simulink library "components_lib"  (Simulink 6.2)
undefined symbols (not defined in the file): A_ang_c, A_att_c, A_est, A_kalman, albedo_onboard_wrapper, B_ang_c, B_att_c, B_est, B_kalman, C_ang_c, C_att_c, C_est, C_i, C_kalman, C_p, Cd, D_ang_c, D_att_c, D_est, D_kalman, Dim, DiscIntNeverNeededParam, Hr, Hs, inerti, Ki, Kr, Ks, magnitude, otoquest, otoquest_with_pro, qmethod, rho, sat_temp_start, ss_proj3, sun_emu_angles2currents, sun_emu_vec2angles, Ts, vector_projection_onto_plane, w_mw_i, w_mw_init, zenith2ref
libraries: components_lib x163, simulink x44, albedo_lib x4, Accessories_lib x3, simulink_extras x2, discrete_bdot_filter x1
(part 2 of 5)

== system components_lib/Disturbances/Gravity ==
  R_m(I) : Inport  Port=1  LatchInput=off
  R_s(I) : Inport  Port=2  LatchInput=off
  R_sc(I) : Inport  Port=3  LatchInput=off
  I(C) : Inport  Port=4  LatchInput=off
  "q(I -> S)" : Inport  Port=5  LatchInput=off
  q(C->S) : Inport  Port=6  LatchInput=off
  M_sat : Inport  Port=7  LatchInput=off
  Gain : Gain  Gain=-1  SaturateOnIntegerOverflow=on
  Gravity Gradient Torque : Subsystem
  Gravity Moon : Subsystem
  Gravity Sun : Subsystem
  Product : Product  SaturateOnIntegerOverflow=on
  Sum : Sum  Inputs=+++  SaturateOnIntegerOverflow=on
  Sum1 : Sum  Inputs=|+-  SaturateOnIntegerOverflow=on
  Sum2 : Sum  Inputs=|+-  SaturateOnIntegerOverflow=on
  Zonal Harmonics  Earth : Subsystem
  N_gr(S) : Outport
  F_gr(I) : Outport  Port=2
  wires:
  Gain/1 -> Product/1
  Gravity Sun/1(F_s(I)) -> Sum/2
  Gravity Moon/1(F_m(I)) -> Sum/1
  Sum1/1 -> Gravity Moon/1(R_m_sat(I))
  Sum2/1 -> Gravity Sun/2(R_s_sat(I))
  R_s(I)/1 -> Sum2/1
  R_m(I)/1 -> Sum1/1
  Product/1 -> Sum/3
  Zonal Harmonics  Earth/1(grad(U_zonal(I))) -> Product/2
  Sum/1 -> F_gr(I)/1
  M_sat/1 -> Gain/1, Gravity Sun/1(M_sat), Gravity Moon/2(M_sat)
  Gravity Gradient Torque/1(N_gr(S)) -> N_gr(S)/1
  "q(I -> S)"/1 -> Gravity Gradient Torque/4(q(I->S))
  q(C->S)/1 -> Gravity Gradient Torque/3(q(C->S))
  I(C)/1 -> Gravity Gradient Torque/2(I(C))
  R_sc(I)/1 -> Sum1/2, Sum2/2, Zonal Harmonics  Earth/1(R_sat(I)), Gravity Gradient Torque/1(R_sc(I))

== system components_lib/Disturbances/Magnetic residual disturbance ==
  "Magnetic electronics dipole, d in(S)" : Inport  Port=1  LatchInput=off
  Attitude q(I->S) : Inport  Port=2  LatchInput=off
  Earth rotation q(I->E) : Inport  Port=3  LatchInput=off
  Magnetic field B(E) : Inport  Port=4  LatchInput=off
  Magnetic field E->S : Subsystem
  cross product : Stateflow chart
  N_mres(S) : Outport
  wires:
  "Magnetic electronics dipole, d in(S)"/1 -> cross product/1(u)
  Magnetic field E->S/1(B(S)) -> cross product/2(v)
  cross product/1(y) -> N_mres(S)/1
  Earth rotation q(I->E)/1 -> Magnetic field E->S/2(q(I->E))
  Magnetic field B(E)/1 -> Magnetic field E->S/3(B(E))
  Attitude q(I->S)/1 -> Magnetic field E->S/1(q(I->S))

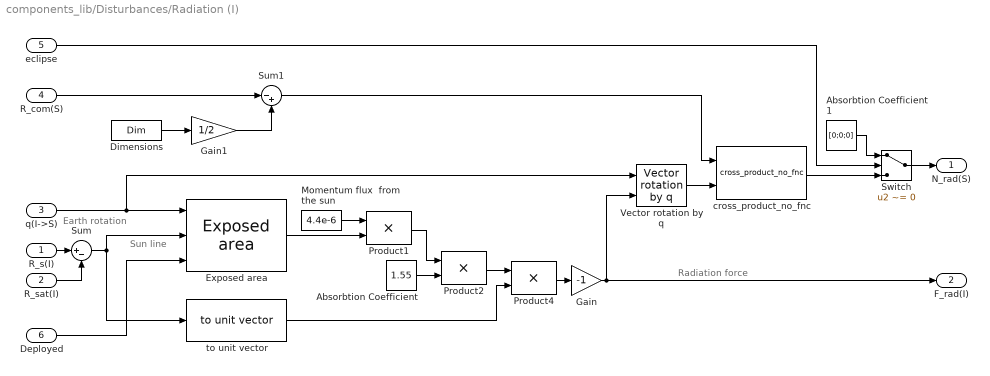
== system components_lib/Disturbances/Radiation (I) ==
  note: Sun line
  note: Earth rotation
  note: Radiation force
  R_s(I) : Inport  Port=1  LatchInput=off
  R_sat(I) : Inport  Port=2  LatchInput=off
  q(I->S) : Inport  Port=3  LatchInput=off
  R_com(S) : Inport  Port=4  LatchInput=off
  eclipse : Inport  Port=5  LatchInput=off
  Deployed : Inport  Port=6  LatchInput=off
  Absorbtion Coefficient : Constant  Value=1.55
  Absorbtion Coefficient1 : Constant  Value=[0;0;0]
  Dimensions : Constant  Value=Dim
  Exposed area : components_lib/Disturbances/Exposed area  dim_sat_area=Dim  dim_sat_array=[-0.30,-0.30]
  Gain : Gain  Gain=-1  SaturateOnIntegerOverflow=on
  Gain1 : Gain  Gain=1/2  SaturateOnIntegerOverflow=on
  Momentum flux  from the sun : Constant  Value=4.4e-6
  Product1 : Product  SaturateOnIntegerOverflow=on
  Product2 : Product  SaturateOnIntegerOverflow=on
  Product4 : Product  SaturateOnIntegerOverflow=on
  Sum : Sum  Inputs=|+-  SaturateOnIntegerOverflow=on
  Sum1 : Sum  Inputs=|-+
  Switch : Switch  Criteria=u2 ~= 0
  Vector rotation by q : components_lib/Math utilities/Quaternion operations/Vector rotation by q
  cross_product_no_fnc : components_lib/Math utilities/Vector operations/cross_product_no_fnc
  to unit vector : components_lib/Math utilities/Vector operations/to unit vector
  N_rad(S) : Outport
  F_rad(I) : Outport  Port=2
  wires:
  Absorbtion Coefficient1/1 -> Switch/1
  Switch/1 -> N_rad(S)/1
  R_s(I)/1 -> Sum/1
  R_sat(I)/1 -> Sum/2
  q(I->S)/1 -> Vector rotation by q/1, Exposed area/1
  Sum/1 -> to unit vector/1, Exposed area/2
  Product1/1 -> Product2/1
  Absorbtion Coefficient/1 -> Product2/2
  Product2/1 -> Product4/1
  to unit vector/1 -> Product4/2
  Product4/1 -> Gain/1
  Gain/1 -> F_rad(I)/1, Vector rotation by q/2
  Vector rotation by q/1 -> cross_product_no_fnc/2
  Exposed area/1 -> Product1/2
  Momentum flux  from the sun/1 -> Product1/1
  cross_product_no_fnc/1 -> Switch/3
  eclipse/1 -> Switch/2
  Dimensions/1 -> Gain1/1
  R_com(S)/1 -> Sum1/1
  Gain1/1 -> Sum1/2
  Sum1/1 -> cross_product_no_fnc/1
  Deployed/1 -> Exposed area/3

== system components_lib/Dynamics and Kinematics/Spacecraft Dynamics ==
  Initial angular velocity W_i(S) : Inport  Port=1  LatchInput=off
  Initial attitude q(I->S) : Inport  Port=2  LatchInput=off
  Controller frame  q(S->C) : Inport  Port=3  LatchInput=off
  Spacecraft Inertia I(C) : Inport  Port=4  LatchInput=off
  N_mt(S) : Inport  Port=5  LatchInput=off
  N_mw(S) : Inport  Port=6  LatchInput=off
  H_mw(S) : Inport  Port=7  LatchInput=off
  Disturbance N_dist(S) : Inport  Port=8  LatchInput=off
  deployed : Inport  Port=9  LatchInput=off
  Inertia deployed I_d(C) : Inport  Port=10  LatchInput=off
  Reverse quaternion rotation : components_lib/Math utilities/Quaternion operations/Reverse quaternion rotation
  Rotation of q1 by q1 : components_lib/Math utilities/Quaternion operations/Rotation of q1 by q2
  Rotation of q1 by q2 : components_lib/Math utilities/Quaternion operations/Rotation of q1 by q2
  Sum : Sum  Inputs=+++  SaturateOnIntegerOverflow=on
  Switch : Switch  Criteria=u2 > Threshold
  Vector rotation by q{,1..3} (4 alike) : components_lib/Math utilities/Vector operations/Vector rotation by q
  sc-dynamics : S-Function  FunctionName=scdynamics
  w to q : components_lib/Math utilities/Quaternion operations/w to q
  Attitude q(I->S) : Outport
  Angular velocity W(S) : Outport  Port=2
  wires:
  N_mw(S)/1 -> Sum/1
  Disturbance N_dist(S)/1 -> Sum/3
  N_mt(S)/1 -> Sum/2
  Vector rotation by q1/1 -> sc-dynamics/2
  Rotation of q1 by q1/1 -> Attitude q(I->S)/1
  sc-dynamics/1 -> Vector rotation by q3/2, w to q/1
  H_mw(S)/1 -> Vector rotation by q2/2
  w to q/1 -> Rotation of q1 by q1/1
  Rotation of q1 by q2/1 -> w to q/2
  Vector rotation by q3/1 -> Angular velocity W(S)/1
  Reverse quaternion rotation/1 -> Vector rotation by q3/1, Rotation of q1 by q1/2
  Vector rotation by q2/1 -> sc-dynamics/3
  Vector rotation by q/1 -> sc-dynamics/1
  Initial attitude q(I->S)/1 -> Rotation of q1 by q2/1
  Controller frame  q(S->C)/1 -> Vector rotation by q/1, Rotation of q1 by q2/2, Vector rotation by q1/1, Reverse quaternion rotation/1, Vector rotation by q2/1
  Initial angular velocity W_i(S)/1 -> Vector rotation by q/2
  Sum/1 -> Vector rotation by q1/2
  Switch/1 -> sc-dynamics/4
  Inertia deployed I_d(C)/1 -> Switch/1
  Spacecraft Inertia I(C)/1 -> Switch/3
  deployed/1 -> Switch/2

== system components_lib/Math utilities/Quaternion operations ==
  Quarternion error : Subsystem
  Quaternion inverter : Subsystem
  Quaternion mulitiplication : S-Function  FunctionName=qmul
  Reverse quaternion rotation : Subsystem
  Rotation from q1 to q2 : Subsystem
  Rotation of q1 by q2 : Subsystem
  Vector rotation by q : Subsystem
  qmul no func : Subsystem
  quaternion composition : Subsystem
  quaternion decomposition : Subsystem
  quaternion expansion : Subsystem
  quaternion2euler : Subsystem
  w to q : Subsystem
  ||q|| : Subsystem

== system components_lib/Math utilities/Vector operations ==
  Projection of a onto b : Subsystem
  Vector rotation by q : Subsystem
  cross_product : Subsystem
  cross_product_no_fnc : Subsystem
  modulus : Subsystem
  norm : Subsystem
  pow : Subsystem  Description=u^v
  sign : Subsystem
  to unit vector : Subsystem
  vector projection onto plane : Subsystem
  ||V|| : MATLABFcn  MATLABFcn=norm

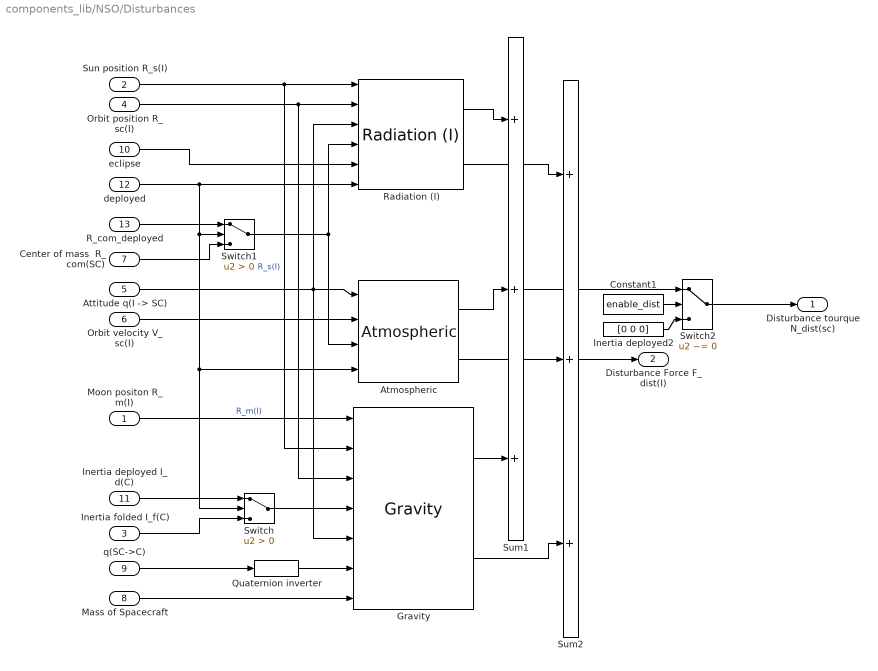
== system components_lib/NSO/Disturbances ==
  Moon positon R_m(I) : Inport  Port=1  LatchInput=off
  Sun position R_s(I) : Inport  Port=2  LatchInput=off
  Inertia folded I_f(C) : Inport  Port=3  LatchInput=off
  Orbit position R_sc(I) : Inport  Port=4  LatchInput=off
  "Attitude q(I -> SC)" : Inport  Port=5  LatchInput=off
  Orbit velocity V_sc(I) : Inport  Port=6  LatchInput=off
  Center of mass  R_com(SC) : Inport  Port=7  LatchInput=off
  "Mass of Spacecraft " : Inport  Port=8  LatchInput=off
  q(SC->C) : Inport  Port=9  LatchInput=off
  eclipse : Inport  Port=10  LatchInput=off
  Inertia deployed I_d(C) : Inport  Port=11  LatchInput=off
  deployed : Inport  Port=12  LatchInput=off
  R_com_deployed : Inport  Port=13  LatchInput=off
  Atmospheric : components_lib/Disturbances/Atmospheric
  Constant1 : Constant  Value=enable_dist
  Gravity : components_lib/Disturbances/Gravity  G=6.673e-11  M_sun=1.98892e30  M_moon=7.36e22  M_earth=5.9742e24
  Inertia deployed2 : Constant  Value=[0 0 0]
  Quaternion inverter : components_lib/Math utilities/Quaternion operations/Quaternion inverter
  Radiation (I) : components_lib/Disturbances/Radiation (I)
  Sum1 : Sum  Inputs=+++  SaturateOnIntegerOverflow=on
  Sum2 : Sum  Inputs=+++  SaturateOnIntegerOverflow=on
  Switch : Switch  Criteria=u2 > Threshold
  Switch1 : Switch  Criteria=u2 > Threshold
  Switch2 : Switch  Criteria=u2 ~= 0
  Disturbance tourque N_dist(sc) : Outport
  Disturbance Force F_dist(I) : Outport  Port=2
  wires:
  deployed/1 -> Radiation (I)/6, Atmospheric/4, Switch/2, Switch1/2
  Switch/1 -> Gravity/4
  Inertia deployed I_d(C)/1 -> Switch/1
  Inertia folded I_f(C)/1 -> Switch/3
  eclipse/1 -> Radiation (I)/5
  Sum2/1 -> Disturbance Force F_dist(I)/1
  Sum1/1 -> Switch2/1
  Gravity/2 -> Sum2/3
  Atmospheric/2 -> Sum2/2
  Radiation (I)/2 -> Sum2/1
  Gravity/1 -> Sum1/3
  Atmospheric/1 -> Sum1/2
  Radiation (I)/1 -> Sum1/1
  Orbit velocity V_sc(I)/1 -> Atmospheric/2
  Orbit position R_sc(I)/1 -> Radiation (I)/2, Gravity/3
  "Attitude q(I -> SC)"/1 -> Gravity/5, Radiation (I)/3, Atmospheric/1
  Sun position R_s(I)/1 -> Radiation (I)/1, Gravity/2  "R_s(I)"
  Moon positon R_m(I)/1 -> Gravity/1  "R_m(I)"
  "Mass of Spacecraft "/1 -> Gravity/7
  Quaternion inverter/1 -> Gravity/6
  q(SC->C)/1 -> Quaternion inverter/1
  Center of mass  R_com(SC)/1 -> Switch1/3
  R_com_deployed/1 -> Switch1/1
  Switch1/1 -> Radiation (I)/4, Atmospheric/3
  Inertia deployed2/1 -> Switch2/3
  Constant1/1 -> Switch2/2
  Switch2/1 -> Disturbance tourque N_dist(sc)/1

== system components_lib/NSO/Spacecraft Dynamics ==
  Initial angular velocity W_i(S) : Inport  Port=1  LatchInput=off
  Initial attitude q(I->S) : Inport  Port=2  LatchInput=off
  Controller frame  q(S->C) : Inport  Port=3  LatchInput=off
  Spacecraft Inertia I(C) : Inport  Port=4  LatchInput=off
  N_mt(S) : Inport  Port=5  LatchInput=off
  N_mw(S) : Inport  Port=6  LatchInput=off
  H_mw(S) : Inport  Port=7  LatchInput=off
  Disturbance N_dist(S) : Inport  Port=8  LatchInput=off
  deployed : Inport  Port=9  LatchInput=off
  Inertia deployed I_d(C) : Inport  Port=10  LatchInput=off
  Reverse quaternion rotation : components_lib/Math utilities/Quaternion operations/Reverse quaternion rotation
  Rotation of q1 by q1 : components_lib/Math utilities/Quaternion operations/Rotation of q1 by q2
  Rotation of q1 by q2 : components_lib/Math utilities/Quaternion operations/Rotation of q1 by q2
  Sum : Sum  Inputs=-++  SaturateOnIntegerOverflow=on
  Switch : Switch  Criteria=u2 > Threshold
  Vector rotation by q{,1..3} (4 alike) : components_lib/Math utilities/Vector operations/Vector rotation by q
  sc-dynamics : S-Function  FunctionName=scdynamics
  w to q : components_lib/Math utilities/Quaternion operations/w to q
  Attitude q(I->S) : Outport
  Angular velocity W(S) : Outport  Port=2
  wires:
  N_mw(S)/1 -> Sum/1
  Disturbance N_dist(S)/1 -> Sum/3
  N_mt(S)/1 -> Sum/2
  Vector rotation by q1/1 -> sc-dynamics/2
  Rotation of q1 by q1/1 -> Attitude q(I->S)/1
  sc-dynamics/1 -> Vector rotation by q3/2, w to q/1
  H_mw(S)/1 -> Vector rotation by q2/2
  w to q/1 -> Rotation of q1 by q1/1
  Rotation of q1 by q2/1 -> w to q/2
  Vector rotation by q3/1 -> Angular velocity W(S)/1
  Reverse quaternion rotation/1 -> Vector rotation by q3/1, Rotation of q1 by q1/2
  Vector rotation by q2/1 -> sc-dynamics/3
  Vector rotation by q/1 -> sc-dynamics/1
  Initial attitude q(I->S)/1 -> Rotation of q1 by q2/1
  Controller frame  q(S->C)/1 -> Vector rotation by q/1, Rotation of q1 by q2/2, Vector rotation by q1/1, Reverse quaternion rotation/1, Vector rotation by q2/1
  Initial angular velocity W_i(S)/1 -> Vector rotation by q/2
  Sum/1 -> Vector rotation by q1/2
  Switch/1 -> sc-dynamics/4
  Inertia deployed I_d(C)/1 -> Switch/1
  Spacecraft Inertia I(C)/1 -> Switch/3
  deployed/1 -> Switch/2

== system components_lib/Orbit and Ephemeris/(IGRF) Magnetic field ==
  Spacecraft position R_sc(I) : Inport  Port=1  LatchInput=off
  Earth rotation q(I->E) : Inport  Port=2  LatchInput=off
  Enable : EnablePort
  Magnetic field model : components_lib/Orbit and Ephemeris/Magnetic field model
  T->Gauss : Gain  Gain=1e4  SaturateOnIntegerOverflow=on
  Vector rotation by q : components_lib/Math utilities/Vector operations/Vector rotation by q
  Magnetic field vector B(E) : Outport
  wires:
  T->Gauss/1 -> Magnetic field vector B(E)/1
  Magnetic field model/1 -> T->Gauss/1  "B(I / E)"
  Vector rotation by q/1 -> Magnetic field model/1
  Earth rotation q(I->E)/1 -> Vector rotation by q/1
  Spacecraft position R_sc(I)/1 -> Vector rotation by q/2

== system components_lib/Orbit and Ephemeris/Albedo ==
  Sunlight vector(I) : Inport  Port=1  LatchInput=off
  Nadir vector (I) : Inport  Port=2  LatchInput=off
  q(I>E) : Inport  Port=3  LatchInput=off
  Enable : EnablePort
  Earth Albedo Model : albedo_lib/Earth Albedo Model  eprdata=load('lib/space_environment_emulation/albedo/toolbox/epr_data/2003/ga030101-031231')  redfac=1  Ts=10  enable=on
  Vector rotation by q1 : components_lib/Math utilities/Vector operations/Vector rotation by q
  Vector rotation by q2 : components_lib/Math utilities/Vector operations/Vector rotation by q
  Reflectivity matrix : Outport
  wires:
  Sunlight vector(I)/1 -> Vector rotation by q2/2
  q(I>E)/1 -> Vector rotation by q2/1, Vector rotation by q1/1
  Nadir vector (I)/1 -> Vector rotation by q1/2
  Earth Albedo Model/1 -> Reflectivity matrix/1
  Vector rotation by q2/1 -> Earth Albedo Model/2
  Vector rotation by q1/1 -> Earth Albedo Model/1

== system components_lib/Orbit and Ephemeris/Albedo emulation model ==
  Sunlight vector(I) : Inport  Port=1  LatchInput=off
  Nadir vector (I) : Inport  Port=2  LatchInput=off
  q(I>E) : Inport  Port=3  LatchInput=off
  Earth Albedo Model1 : albedo_lib/Earth Albedo Model  eprdata=mean_epr  redfac=1  Ts=60  enable=on
  Vector rotation by q1 : components_lib/Math utilities/Vector operations/Vector rotation by q
  Vector rotation by q2 : components_lib/Math utilities/Vector operations/Vector rotation by q
  Reflectivity matrix : Outport
  wires:
  Vector rotation by q1/1 -> Earth Albedo Model1/1
  Vector rotation by q2/1 -> Earth Albedo Model1/2
  Earth Albedo Model1/1 -> Reflectivity matrix/1
  Nadir vector (I)/1 -> Vector rotation by q1/2
  q(I>E)/1 -> Vector rotation by q1/1, Vector rotation by q2/1
  Sunlight vector(I)/1 -> Vector rotation by q2/2

== system components_lib/Orbit and Ephemeris/Eclipse model ==
  note: theta_e
  Sun vector (I) : Inport  Port=1  LatchInput=off
  Satellite (I) : Inport  Port=2  LatchInput=off
  Constant : Constant  Value=pi
  Divide : Product  Inputs=*/  OutScaling=2^-10
  Dot Product : simulink/Math Operations/Dot Product  InputSameDT=on  OutDataType=sfix(16)  OutScaling=2^-10  DoSatur=off
  Dot Product1 : simulink/Math Operations/Dot Product  InputSameDT=on  OutDataType=sfix(16)  OutScaling=2^-10  DoSatur=off
  Earth radius : Constant  Value=r_e
  False : Constant  Value=0
  Manual Switch : simulink/Signal Routing/Manual Switch  sw=0  action=0
  Math Function : Math  Operator=sqrt  SaturateOnIntegerOverflow=on
  Max angle : Constant  Value=theta_e/180*pi
  Satellite unit vector : components_lib/Math utilities/Vector operations/to unit vector
  Sum : Sum  Orientation=down  Inputs=-+|
  Sum1 : Sum  Inputs=+-|
  Sun unit vector : components_lib/Math utilities/Vector operations/to unit vector
  Switch : Switch
  Trigonometric Function : Trigonometry  Operator=asin
  Trigonometric Function1 : Trigonometry  Operator=acos
  True : Constant
  "Eclipse: 1 = true, 0 = false" : Outport  PortDimensions=1
  wires:
  Sun vector (I)/1 -> Sun unit vector/1
  Satellite (I)/1 -> Satellite unit vector/1, Dot Product1/1, Dot Product1/2
  Sun unit vector/1 -> Dot Product/1
  Satellite unit vector/1 -> Dot Product/2
  Dot Product/1 -> Trigonometric Function1/1
  Earth radius/1 -> Divide/1
  Math Function/1 -> Divide/2
  Divide/1 -> Trigonometric Function/1
  Trigonometric Function1/1 -> Sum/1
  Constant/1 -> Sum/2
  Sum/1 -> Sum1/1  "theta"
  Sum1/1 -> Switch/2
  True/1 -> Switch/3
  False/1 -> Switch/1
  Switch/1 -> "Eclipse: 1 = true, 0 = false"/1
  Manual Switch/1 -> Sum1/2
  Trigonometric Function/1 -> Manual Switch/2
  Max angle/1 -> Manual Switch/1
  Dot Product1/1 -> Math Function/1

== system components_lib/Orbit and Ephemeris/Ephemeris ==
  Time t(JD) : Inport  Port=1  LatchInput=off
  ECEF : Subsystem
  Moon Position : Subsystem
  Sun Position : Subsystem
  Moon position R_m(I) : Outport
  Sun Position R_s(I) : Outport  Port=2
  Earth Rotation q(I->E) : Outport  Port=3
  wires:
  ECEF/1(q(I->E)) -> Earth Rotation q(I->E)/1  "q(I -> E)"
  Time t(JD)/1 -> Moon Position/1(t(JD)1), Sun Position/1(t(JD)), ECEF/1(t(JD))  "t"
  Moon Position/1(R_m(I)) -> Moon position R_m(I)/1  "R_m(I)"
  Sun Position/1(R_s(I)) -> Sun Position R_s(I)/1  "R_s(I)"

== system components_lib/Orbit and Ephemeris/Magnetic field model ==
  R_sc(E) : Inport  Port=1  LatchInput=off
  S-Function : S-Function  FunctionName=igrfS  Parameters=2002,10
  B(E) : Outport
  wires:
  R_sc(E)/1 -> S-Function/1
  S-Function/1 -> B(E)/1

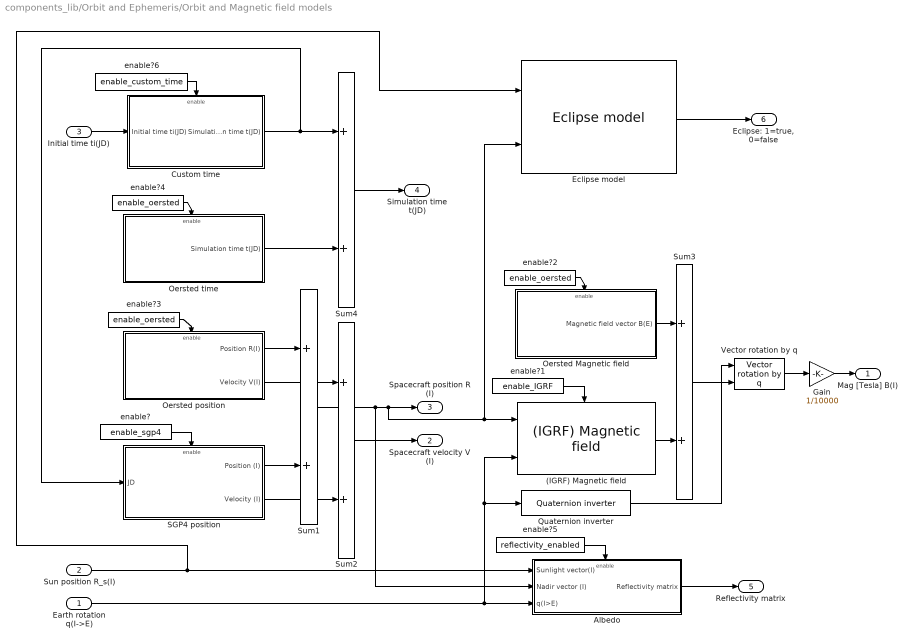
== system components_lib/Orbit and Ephemeris/Orbit and Magnetic field models ==
  Earth rotation q(I->E) : Inport  Port=1  LatchInput=off
  Sun position R_s(I) : Inport  Port=2  LatchInput=off
  Initial time ti(JD) : Inport  Port=3  LatchInput=off
  (IGRF) Magnetic field : components_lib/Orbit and Ephemeris/(IGRF) Magnetic field
  Albedo : Subsystem  AncestorBlock=components_lib/Orbit and Ephemeris/Albedo  TreatAsAtomicUnit=on
  Custom time : Subsystem  TreatAsAtomicUnit=on
  Eclipse model : components_lib/Orbit and Ephemeris/Eclipse model  r_e=6371010  theta_e=65
  Gain : Gain  Gain=1/10000
  Oersted Magnetic field : Subsystem  TreatAsAtomicUnit=on
  Oersted position : Subsystem  TreatAsAtomicUnit=on
  Oersted time : Subsystem  TreatAsAtomicUnit=on
  Quaternion inverter : components_lib/Math utilities/Quaternion operations/Quaternion inverter
  SGP4 position : Subsystem  TreatAsAtomicUnit=on
  Sum{1..4} (4 alike) : Sum
  Vector rotation by q : components_lib/Math utilities/Quaternion operations/Vector rotation by q
  enable? : Constant  Value=enable_sgp4
  enable?1 : Constant  Value=enable_IGRF
  enable?2 : Constant  Value=enable_oersted
  enable?3 : Constant  Value=enable_oersted
  enable?4 : Constant  Value=enable_oersted
  enable?5 : Constant  Value=reflectivity_enabled
  enable?6 : Constant  Value=enable_custom_time
  Mag [Tesla] B(I) : Outport
  Spacecraft velocity V (I) : Outport  Port=2
  Spacecraft position R (I) : Outport  Port=3
  Simulation time t(JD) : Outport  Port=4
  Reflectivity matrix : Outport  Port=5
  "Eclipse: 1=true, 0=false" : Outport  Port=6  PortDimensions=1
  wires:
  Gain/1 -> Mag [Tesla] B(I)/1
  Sum3/1 -> Vector rotation by q/2
  (IGRF) Magnetic field/1 -> Sum3/2
  Oersted Magnetic field/1(Magnetic field vector B(E)) -> Sum3/1
  Sum2/1 -> Spacecraft velocity V (I)/1
  Sum1/1 -> Spacecraft position R (I)/1, Eclipse model/2, (IGRF) Magnetic field/1, Albedo/2(Nadir vector (I))
  SGP4 position/2(Velocity (I)) -> Sum2/2
  Oersted position/2(Velocity V(I)) -> Sum2/1
  SGP4 position/1(Position (I)) -> Sum1/2
  Oersted position/1(Position R(I)) -> Sum1/1
  enable?4/1 -> Oersted time/Enable
  enable?/1 -> SGP4 position/Enable
  Earth rotation q(I->E)/1 -> Quaternion inverter/1, (IGRF) Magnetic field/2, Albedo/3(q(I>E))
  Sun position R_s(I)/1 -> Eclipse model/1, Albedo/1(Sunlight vector(I))
  Albedo/1(Reflectivity matrix) -> Reflectivity matrix/1
  enable?3/1 -> Oersted position/Enable
  Initial time ti(JD)/1 -> Custom time/1(Initial time ti(JD))
  Oersted time/1(Simulation time t(JD)) -> Sum4/2
  Custom time/1(Simulation time t(JD)) -> Sum4/1, SGP4 position/1(JD)
  Sum4/1 -> Simulation time t(JD)/1
  enable?6/1 -> Custom time/Enable
  Quaternion inverter/1 -> Vector rotation by q/1
  Vector rotation by q/1 -> Gain/1
  enable?1/1 -> (IGRF) Magnetic field/Enable
  enable?2/1 -> Oersted Magnetic field/Enable
  enable?5/1 -> Albedo/Enable
  Eclipse model/1 -> "Eclipse: 1=true, 0=false"/1

== system components_lib/Other model utilities/AAUSAT-II Animation ==
  SC position : Inport  Port=1  LatchInput=off
  SC quaternion : Inport  Port=2  LatchInput=off
  SC veloc : Inport  Port=3  LatchInput=off
  sun vector(I) : Inport  Port=4  LatchInput=off
  Earth rotation : Inport  Port=5  LatchInput=off
  Mux3 : Mux  Inputs=5
  S-Function : S-Function  FunctionName=aausatanim  Parameters=Config
  wires:
  Mux3/1 -> S-Function/1
  SC position/1 -> Mux3/1
  SC quaternion/1 -> Mux3/2
  sun vector(I)/1 -> Mux3/4
  Earth rotation/1 -> Mux3/5
  SC veloc/1 -> Mux3/3

== system components_lib/Sensor Emulation/Emulation of gyros ==
  W(S) [rad/s] : Inport  Port=1  LatchInput=off
  Temperature [K] : Inport  Port=2  LatchInput=off
  Amplification and ADC : Subsystem
  Demux : Demux  Outputs=3
  Demux1 : Demux  Outputs=3
  Gain : Gain  Gain=-1
  Gyro sensor block : Subsystem
  Mux : Mux  Inputs=6
  V_ADC [mV] : Outport
  wires:
  Amplification and ADC/1(V_discrete) -> V_ADC [mV]/1
  Demux/3 -> Mux/6
  Demux/2 -> Mux/5
  Demux/1 -> Mux/4
  Demux1/3 -> Mux/3
  Demux1/2 -> Mux/2
  Demux1/1 -> Mux/1
  Gain/1 -> Demux/1
  W(S) [rad/s]/1 -> Gain/1, Demux1/1
  Mux/1 -> Gyro sensor block/1(W(S) [rad/s])
  Temperature [K]/1 -> Gyro sensor block/2(Temperature [K])
  Gyro sensor block/1(W_sens(S) [mV]) -> Amplification and ADC/1(V_cont)

== system components_lib/Sensor Emulation/Emulation of magnetometer ==
  B(I) : Inport  Port=1  LatchInput=off
  q(I->S) : Inport  Port=2  LatchInput=off
  Temperature  [K] : Inport  Port=3  LatchInput=off
  Amplification and ADC : Subsystem
  magnetometer sensor block : Subsystem
  V_ADC [mV] : Outport
  wires:
  magnetometer sensor block/1(Voltage  [mV]) -> Amplification and ADC/1(V_cont)
  Amplification and ADC/1(V_discrete) -> V_ADC [mV]/1
  B(I)/1 -> magnetometer sensor block/1(B(I))
  q(I->S)/1 -> magnetometer sensor block/2(q(I->S))
  Temperature  [K]/1 -> magnetometer sensor block/3(Temperature  [K])

== system components_lib/Sensor Emulation/Emulation of temperature sensors ==
  Band-Limited White Noise : simulink/Sources/Band-Limited White Noise  Cov=1e-9  Ts=1  seed=33232
  Constant : Constant  Value=sat_temp_start
  Sum : Sum  Inputs=|++
  Temperature_meas [mV] : Outport
  Temperature [K] : Outport  Port=2
  wires:
  Sum/1 -> Temperature_meas [mV]/1
  Constant/1 -> Sum/1, Temperature [K]/1
  Band-Limited White Noise/1 -> Sum/2

== system components_lib/Sensor Emulation/Sensor Emulation ==
  Attitude q(I->S) : Inport  Port=1  LatchInput=off
  Mag. field B(I) : Inport  Port=2  LatchInput=off
  Sun pos. R_s(I) : Inport  Port=3  LatchInput=off
  Earth rot. q(I->E) : Inport  Port=4  LatchInput=off
  Ang. vel. W(S) : Inport  Port=5  LatchInput=off
  S/C pos. R_sa(I) : Inport  Port=6  LatchInput=off
  Reflectivity matrix : Inport  Port=7  LatchInput=off
  Eclipse sim : Inport  Port=8  LatchInput=off
  Enable : EnablePort
  Emulation of gyros : components_lib/Sensor Emulation/Emulation of gyros  scale_model=[859.4 859.4 859.4 859.4 859.4 859.4]  offset_model=[2500 2500 2500 2500 2500 2500]  e_bias=[0.0012 0.0012 0.0012 0.0012 0.0012 0.0012]  e_align=[1 1 1 1 1 1]  e_scale=[0.1 0.1 0.1 0.1 0.1 0.1]  e_noise=[0.0035 0.0035 0.0035 0.0035 0.0035 0.0035]*1e-6  e_noise_seed=[23341 43534 43433 22299 32478 21932]  e_drift_scale_model=[0.075 0.075 0.075 0.075 0.075 0.075]  e_drift_offset_model=[0.012 0.012 0.012 0.012 0.012 0.012]  op_amp_gain=[10 10 10 10 10 10]  op_amp_offset=[2500 2500 2500 2500 2500 2500]
  Emulation of magnetometer : components_lib/Sensor Emulation/Emulation of magnetometer  v_supply_model=5  sens_model=[1 1 1]  e_drift_sens_model=[-3000 -3000 -3000]  e_scale=[0.05 0.05 0.05]  e_align=1*0  e_orth=1*0  e_noise=[32 32 32]*1e-6*0  e_noise_seed=[23341 43534 43433]  op_amp_gain=[500 500 500]  op_amp_offset=[2500 2500 2500]
  Emulation of temperature sensors : components_lib/Sensor Emulation/Emulation of temperature sensors
  Sun sensors : components_lib/Sensor Emulation/Sun sensors  sun_flux=1366.9  alpha_align=[1 1 1 1 2 2]*0  temp_drift=0.00233  sigma_noise=0.0000014*0  noise_seed=[0.0000008 0.0000011 0.0000004 0.0000005 0.0000000 0.0000002]*0  op_amp_gain=1  op_amp_offset=0
  Magnotometer (S)  V_ADC [mV] : Outport
  Gyros  (S) V_ADC [mV] : Outport  Port=2
  Sun sensors (S)  [mA] : Outport  Port=3
  Temperature (S) V_ADC [mV] : Outport  Port=4
  wires:
  Mag. field B(I)/1 -> Emulation of magnetometer/1
  Attitude q(I->S)/1 -> Emulation of magnetometer/2, Sun sensors/4
  Earth rot. q(I->E)/1 -> Sun sensors/5
  Emulation of magnetometer/1 -> Magnotometer (S)  V_ADC [mV]/1
  Ang. vel. W(S)/1 -> Emulation of gyros/1
  Emulation of gyros/1 -> Gyros  (S) V_ADC [mV]/1
  S/C pos. R_sa(I)/1 -> Sun sensors/2
  Sun pos. R_s(I)/1 -> Sun sensors/1
  Sun sensors/1 -> Sun sensors (S)  [mA]/1
  Reflectivity matrix/1 -> Sun sensors/3
  Emulation of temperature sensors/1 -> Temperature (S) V_ADC [mV]/1
  Emulation of temperature sensors/2 -> Emulation of magnetometer/3, Sun sensors/6, Emulation of gyros/2
  Eclipse sim/1 -> Sun sensors/7

== system components_lib/Sensor Emulation/Sun sensors ==
  Sun pos. R_s(I) : Inport  Port=1  LatchInput=off
  S/C pos. R_sa(I) : Inport  Port=2  LatchInput=off
  Reflectivity matrix : Inport  Port=3  LatchInput=off
  q(I->S) : Inport  Port=4  LatchInput=off
  q(I->E) : Inport  Port=5  LatchInput=off
  Temperature  [K] : Inport  Port=6  LatchInput=off
  Eclipse sim : Inport  Port=7  LatchInput=off
  Amplification and ADC : Subsystem
  Frame conversion : Subsystem
  q rot : Scope  NumInputPorts=3
      settings: YMin=-3e+10~-5~-5  YMax=1.5e+11~5~5  SaveName=ScopeData5
  sun sensor model : Subsystem
  Sun_currents [mA] : Outport
  wires:
  Eclipse sim/1 -> sun sensor model/6(Eclipse sim)
  Frame conversion/3(q(S->E)) -> sun sensor model/3(q(S->E))
  q(I->E)/1 -> Frame conversion/4(q(I->E))
  sun sensor model/1(Currents [mA]) -> q rot/3, Amplification and ADC/1(Currents [mA])  "currents"
  Reflectivity matrix/1 -> sun sensor model/4(Reflectivity matrix)
  Temperature  [K]/1 -> sun sensor model/5(Temperature  [K])
  Frame conversion/1(Sun pos. R_s(S)) -> q rot/2, sun sensor model/1(Sun position R_s(S))
  Frame conversion/2(Nadir(E)) -> q rot/1, sun sensor model/2(Nadir(E))  "nadir (E)"
  S/C pos. R_sa(I)/1 -> Frame conversion/2(S/C pos. R_sa(I))
  Sun pos. R_s(I)/1 -> Frame conversion/1(Sun pos. R_s(I))
  q(I->S)/1 -> Frame conversion/3(q(I->S))
  Amplification and ADC/1(I_ADC [mA]) -> Sun_currents [mA]/1

== system components_lib/ACS/Controllers/Angular velocity  controller ==
  omega : Inport  Port=1  LatchInput=off
  omega_ref : Inport  Port=2  LatchInput=off
  State-Space : StateSpace  A=A_ang_c  B=B_ang_c  C=C_ang_c  D=D_ang_c
  Sum : Sum  Inputs=|+-
  N_mw : Outport
  wires:
  omega_ref/1 -> Sum/2
  omega/1 -> Sum/1
  State-Space/1 -> N_mw/1
  Sum/1 -> State-Space/1

== system components_lib/ACS/Controllers/Attitude controller ==
  q_att : Inport  Port=1  LatchInput=off
  q_ref : Inport  Port=2  LatchInput=off
  omega : Inport  Port=3  LatchInput=off
  Mux : Mux  Inputs=2
  Quarternion error : components_lib/Math utilities/Quaternion operations/Quarternion error
  Selector : Selector  Elements=[1 2 3]  InputPortWidth=4
  State-Space : StateSpace  A=A_att_c  B=B_att_c  C=C_att_c  D=D_att_c
  omega_ref : Outport
  wires:
  State-Space/1 -> omega_ref/1
  Quarternion error/1 -> Selector/1
  q_att/1 -> Quarternion error/1
  q_ref/1 -> Quarternion error/2
  Selector/1 -> Mux/1
  omega/1 -> Mux/2
  Mux/1 -> State-Space/1

== system components_lib/ACS/Controllers/Attitude controller with integrator ==
  q_att : Inport  Port=1  LatchInput=off
  q_ref : Inport  Port=2  LatchInput=off
  omega : Inport  Port=3  LatchInput=off
  Integrator : Integrator  LimitOutput=on  UpperSaturationLimit=0.01  LowerSaturationLimit=-0.01
  Mux : Mux  Inputs=3
  Quarternion error : components_lib/Math utilities/Quaternion operations/Quarternion error
  Selector : Selector  Elements=[1 2 3]  InputPortWidth=4
  State-Space : StateSpace  A=A_att_c  B=B_att_c  C=C_att_c  D=D_att_c
  omega_ref : Outport
  wires:
  Mux/1 -> State-Space/1
  omega/1 -> Mux/2
  Selector/1 -> Mux/1, Integrator/1
  q_ref/1 -> Quarternion error/2
  q_att/1 -> Quarternion error/1
  Quarternion error/1 -> Selector/1
  State-Space/1 -> omega_ref/1
  Integrator/1 -> Mux/3

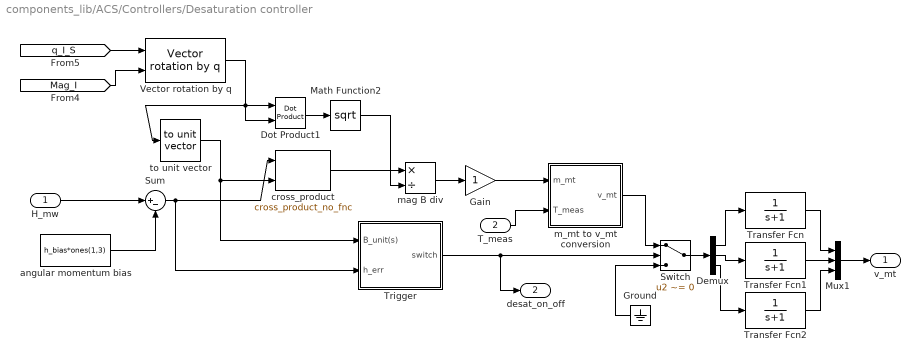
== system components_lib/ACS/Controllers/Desaturation controller ==
  H_mw : Inport  Port=1  LatchInput=off
  T_meas : Inport  Port=2  LatchInput=off
  Demux : Demux  Outputs=3
  Dot Product1 : simulink/Math Operations/Dot Product  InputSameDT=on  OutDataType=sfix(16)  OutScaling=2^-10  DoSatur=off
  Gain : Gain
  Ground : Ground  Orientation=left
  Math Function2 : Math  Operator=sqrt  SaturateOnIntegerOverflow=on
  Mux1 : Mux  Inputs=3
  Sum : Sum  Inputs=|+-
  Switch : Switch  Criteria=u2 ~= 0  Threshold=0.5
  Transfer Fcn : TransferFcn  Denominator=[1 1]
  Transfer Fcn1 : TransferFcn  Denominator=[1 1]
  Transfer Fcn2 : TransferFcn  Denominator=[1 1]
  Trigger : Subsystem
  Vector rotation by q : components_lib/Math utilities/Quaternion operations/Vector rotation by q
  angular momentum bias : Constant  Value=h_bias*ones(1,3)
  cross_product : components_lib/Math utilities/Vector operations/cross_product_no_fnc
  m_mt to v_mt conversion : Subsystem  mask{n_mt=[435 435 865], A_mt=[0.21*0.07 0.21*0.07 0.07*0.07], L_mt=[26.956e-3 26.956e-3 59.256e-3], v_max_mt=5}
      mask prompts: n_mt "Coil winding number [n_x n_y n_z]"; A_mt "Coil area [A_mt_x A_mt_y A_mt_z]"; L_mt "Coil inductance [L_mt_x L_mt_y L_mt_z]"; v_max_mt "Maximum voltage"
  mag B div : Product  Inputs=*/  OutScaling=2^-10
  to unit vector : components_lib/Math utilities/Vector operations/to unit vector
  v_mt : Outport
  desat_on_off : Outport  Port=2
  wires:
  H_mw/1 -> Sum/1
  angular momentum bias/1 -> Sum/2
  [Mag_I] -> Vector rotation by q/2
  [q_I_S] -> Vector rotation by q/1
  Sum/1 -> cross_product/1, Trigger/2(h_err)
  cross_product/1 -> mag B div/1
  Ground/1 -> Switch/3
  T_meas/1 -> m_mt to v_mt conversion/2(T_meas)
  mag B div/1 -> Gain/1
  m_mt to v_mt conversion/1(v_mt) -> Switch/1
  Dot Product1/1 -> Math Function2/1
  Math Function2/1 -> mag B div/2
  Gain/1 -> m_mt to v_mt conversion/1(m_mt)
  Switch/1 -> Demux/1
  Demux/1 -> Transfer Fcn/1
  Demux/2 -> Transfer Fcn1/1
  Demux/3 -> Transfer Fcn2/1
  Transfer Fcn/1 -> Mux1/1
  Transfer Fcn1/1 -> Mux1/2
  Transfer Fcn2/1 -> Mux1/3
  Mux1/1 -> v_mt/1
  Vector rotation by q/1 -> Dot Product1/2, Dot Product1/1, to unit vector/1
  to unit vector/1 -> cross_product/2, Trigger/1(B_unit(s))
  Trigger/1(switch) -> Switch/2, desat_on_off/1

== system components_lib/ACS/Controllers/Detumble controller ==
  q(I->S) : Inport  Port=1  LatchInput=off
  B(I) : Inport  Port=2  LatchInput=off
  Constant : Constant  Value=ctrl
  Continous B-dot controller : Subsystem
  Discrete B-dot controller : Subsystem
  Magnetic field I to S : Subsystem
  Merge : Merge
  Switch Case : SwitchCase  CaseConditions={2,3}  CaseShowDefault=off
  enable/disable continous controller : Subsystem  TreatAsAtomicUnit=on
  enable/disable discrete controller : Subsystem  TreatAsAtomicUnit=on
  m_mt(S) : Outport
  wires:
  Switch Case/1 -> enable/disable continous controller/Action
  enable/disable continous controller/1(Out1) -> Merge/1
  Continous B-dot controller/1(m_mt(S)) -> enable/disable continous controller/1(In1)
  enable/disable discrete controller/1(Out1) -> Merge/2
  Discrete B-dot controller/1(m_mt(s)) -> enable/disable discrete controller/1(In1)
  Merge/1 -> m_mt(S)/1
  Switch Case/2 -> enable/disable discrete controller/Action
  Constant/1 -> Switch Case/1
  Magnetic field I to S/1(B(S)) -> Continous B-dot controller/1(B(S)), Discrete B-dot controller/1(B(S))
  q(I->S)/1 -> Magnetic field I to S/1(q(I->S))
  B(I)/1 -> Magnetic field I to S/2(B(I))

== system components_lib/ACS/Controllers/Estimation of dist Kalman filter ==
  control_torque : Inport  Port=1  LatchInput=off
  omega : Inport  Port=2  LatchInput=off
  Mux : Mux  Inputs=2
  State-Space : StateSpace  A=A_kalman  B=B_kalman  C=C_kalman  D=D_kalman
  estimated disturbance : Outport
  wires:
  omega/1 -> Mux/2
  Mux/1 -> State-Space/1
  control_torque/1 -> Mux/1
  State-Space/1 -> estimated disturbance/1

== system components_lib/ACS/Controllers/Estimation of dist linear filter ==
  control_torque : Inport  Port=1  LatchInput=off
  omega : Inport  Port=2  LatchInput=off
  Mux : Mux  Inputs=2
  State-Space : StateSpace  A=A_est  B=B_est  C=C_est  D=D_est
  estimated disturbance : Outport
  wires:
  State-Space/1 -> estimated disturbance/1
  control_torque/1 -> Mux/1
  Mux/1 -> State-Space/1
  omega/1 -> Mux/2

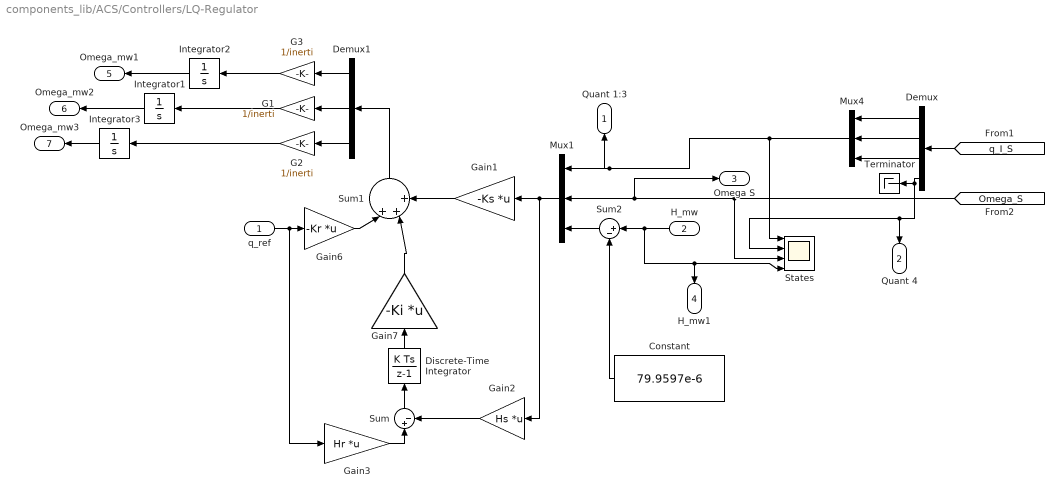
== system components_lib/ACS/Controllers/LQ-Regulator ==
  q_ref : Inport  Port=1  LatchInput=off
  H_mw : Inport  Orientation=left  Port=2  LatchInput=off
  Constant : Constant  Orientation=left  Value=79.9597e-6
  Demux : Demux  Orientation=left
  Demux1 : Demux  Orientation=left  Outputs=3
  Discrete-Time Integrator : DiscreteIntegrator  Orientation=up  SampleTime=Ts  ICPrevOutput=DiscIntNeverNeededParam  ICPrevScaledInput=DiscIntNeverNeededParam
  G1 : Gain  Orientation=left  Gain=1/inerti
  G2 : Gain  Orientation=left  Gain=1/inerti
  G3 : Gain  Orientation=left  Gain=1/inerti
  Gain1 : Gain  Orientation=left  Gain=-Ks  Multiplication=Matrix(K*u)
  Gain2 : Gain  Orientation=left  Gain=Hs  Multiplication=Matrix(K*u)
  Gain3 : Gain  Gain=Hr  Multiplication=Matrix(K*u)
  Gain6 : Gain  Gain=-Kr  Multiplication=Matrix(K*u)
  Gain7 : Gain  Orientation=up  Gain=-Ki  Multiplication=Matrix(K*u)
  Integrator1 : Integrator  Orientation=left  LimitOutput=on  UpperSaturationLimit=576  LowerSaturationLimit=-576
  Integrator2 : Integrator  Orientation=left  LimitOutput=on  UpperSaturationLimit=576  LowerSaturationLimit=-576
  Integrator3 : Integrator  Orientation=left  LimitOutput=on  UpperSaturationLimit=576  LowerSaturationLimit=-576
  Mux1 : Mux  Orientation=left  Inputs=3
  Mux4 : Mux  Orientation=left  Inputs=3
  States : Scope  NumInputPorts=4
      settings: TimeRange=600  YMin=-0.2~0.9225~-0.0125~0  YMax=0.4~0.9475~0.0125~0.00014
  Sum : Sum  Orientation=up  Inputs=|+-
  Sum1 : Sum  Orientation=up  Inputs=|+++
  Sum2 : Sum  Orientation=left  Inputs=|+-
  Terminator : Terminator
  Quant 1:3 : Outport  Orientation=up
  Quant 4 : Outport  Orientation=down  Port=2
  Omega S : Outport  Port=3
  H_mw1 : Outport  Orientation=down  Port=4
  Omega_mw1 : Outport  Orientation=left  Port=5
  Omega_mw2 : Outport  Orientation=left  Port=6
  Omega_mw3 : Outport  Orientation=left  Port=7
  wires:
  Mux1/1 -> Gain1/1, Gain2/1
  Gain2/1 -> Sum/2
  Gain3/1 -> Sum/1
  Sum/1 -> Discrete-Time Integrator/1
  Discrete-Time Integrator/1 -> Gain7/1
  Gain1/1 -> Sum1/3
  Gain7/1 -> Sum1/2
  Gain6/1 -> Sum1/1
  q_ref/1 -> Gain6/1, Gain3/1
  Constant/1 -> Sum2/2
  Sum2/1 -> Mux1/3
  Demux/4 -> Terminator/1, States/2, Quant 4/1
  [q_I_S] -> Demux/1
  Demux/1 -> Mux4/1
  Demux/2 -> Mux4/2
  Demux/3 -> Mux4/3
  [Omega_S] -> States/3, Mux1/2, Omega S/1
  Mux4/1 -> States/1, Mux1/1, Quant 1:3/1
  Sum1/1 -> Demux1/1
  H_mw/1 -> Sum2/1, States/4, H_mw1/1
  G3/1 -> Integrator2/1
  G1/1 -> Integrator1/1
  G2/1 -> Integrator3/1
  Demux1/1 -> G3/1
  Demux1/2 -> G1/1
  Demux1/3 -> G2/1
  Integrator2/1 -> Omega_mw1/1
  Integrator1/1 -> Omega_mw2/1
  Integrator3/1 -> Omega_mw3/1

== system components_lib/ADS/Attitude Determination/EKF using quaternions ==
  q : Inport  Port=1  LatchInput=off
  w : Inport  Port=2  LatchInput=off
  h_mw : Inport  Port=3  LatchInput=off
  N_mt : Inport  Port=4  LatchInput=off
  q0_in : Inport  Port=5  LatchInput=off
  eclipse : Inport  Port=6  LatchInput=off
  Clock : Clock
      settings: Decimation=10
  Demux1 : Demux  Outputs=16
  EKF : MATLABFcn  MATLABFcn=AAUSAT_II_Kalman  OutputDimensions=16  SampleTime=0.1
  Mux1 : Mux  Inputs=3
  Mux2 : Mux  Inputs=8
  Mux3 : Mux
  Mux4 : Mux  Inputs=3
  Mux5 : Mux  Inputs=3
  Step size : Constant  Value=0.1
  q_out : Outport
  w_out : Outport  Port=2
  q_residual : Outport  Port=3
  w_residual : Outport  Port=4
  wires:
  eclipse/1 -> Mux2/8
  q0_in/1 -> Mux2/6
  q/1 -> Mux2/1
  Mux4/1 -> w_out/1
  Mux3/1 -> q_out/1
  N_mt/1 -> Mux2/4
  h_mw/1 -> Mux2/3
  w/1 -> Mux2/2
  Clock/1 -> Mux2/5
  Demux1/4 -> Mux3/4
  Demux1/3 -> Mux3/3
  Demux1/2 -> Mux3/2
  Demux1/1 -> Mux3/1
  Step size/1 -> Mux2/7
  EKF/1 -> Demux1/1
  Mux2/1 -> EKF/1
  Mux1/1 -> q_residual/1
  Mux5/1 -> w_residual/1
  Demux1/8 -> Mux1/1
  Demux1/9 -> Mux1/2
  Demux1/10 -> Mux1/3
  Demux1/5 -> Mux4/1
  Demux1/6 -> Mux4/2
  Demux1/7 -> Mux4/3
  Demux1/11 -> Mux5/1
  Demux1/12 -> Mux5/2
  Demux1/13 -> Mux5/3

== system components_lib/ADS/Attitude Determination/EKF using sun and mag vectors ==
  R_sun(S) : Inport  Port=1  LatchInput=off
  b(S) : Inport  Port=2  LatchInput=off
  w(S) : Inport  Port=3  LatchInput=off
  R_sun(I) : Inport  Port=4  LatchInput=off
  b(I) : Inport  Port=5  LatchInput=off
  h_mw : Inport  Port=6  LatchInput=off
  N_mt : Inport  Port=7  LatchInput=off
  q0 : Inport  Port=8  LatchInput=off
  Eclipse : Inport  Port=9  LatchInput=off
  Clock : Clock
      settings: Decimation=10
  Demux1 : Demux  Outputs=7
  EKF : MATLABFcn  MATLABFcn=AAUSAT_II_Kalman_BS_vectors  OutputDimensions=7  SampleTime=0.1
  Mux2 : Mux  Inputs=11
  Mux3 : Mux
  Mux4 : Mux  Inputs=3
  Step size : Constant  Value=0.1
  q_out : Outport
  w_out : Outport  Port=2
  wires:
  w(S)/1 -> Mux2/3
  Eclipse/1 -> Mux2/11
  Demux1/1 -> Mux3/1
  Demux1/2 -> Mux3/2
  Demux1/3 -> Mux3/3
  Demux1/4 -> Mux3/4
  Mux3/1 -> q_out/1
  Step size/1 -> Mux2/10
  q0/1 -> Mux2/9
  Clock/1 -> Mux2/8
  N_mt/1 -> Mux2/7
  h_mw/1 -> Mux2/6
  b(I)/1 -> Mux2/5
  R_sun(I)/1 -> Mux2/4
  Mux2/1 -> EKF/1
  EKF/1 -> Demux1/1
  Demux1/5 -> Mux4/1
  Demux1/6 -> Mux4/2
  Demux1/7 -> Mux4/3
  R_sun(S)/1 -> Mux2/1
  b(S)/1 -> Mux2/2
  Mux4/1 -> w_out/1

== system components_lib/ADS/Attitude Determination/EKF using sun and mag vectors .. and removing bias ==
  R_sun(S) : Inport  Port=1  LatchInput=off
  b(S) : Inport  Port=2  LatchInput=off
  w(S) : Inport  Port=3  LatchInput=off
  R_sun(I) : Inport  Port=4  LatchInput=off
  b(I) : Inport  Port=5  LatchInput=off
  h_mw : Inport  Port=6  LatchInput=off
  N_mt : Inport  Port=7  LatchInput=off
  q0 : Inport  Port=8  LatchInput=off
  Eclipse : Inport  Port=9  LatchInput=off
  Clock : Clock
      settings: Decimation=10
  EKF : MATLABFcn  MATLABFcn=AAUSAT_II_Kalman_BS_bias_vectors  OutputDimensions=7+12+12  SampleTime=0.1
  Mux2 : Mux  Inputs=11
  Selector : Selector  Elements=(1:4)  InputPortWidth=7+12+12
  Selector1 : Selector  Elements=(5:7)  InputPortWidth=7+12+12
  Selector2 : Selector  Elements=(8:19)  InputPortWidth=7+12+12
  Selector3 : Selector  Elements=(20:31)  InputPortWidth=7+12+12
  Step size : Constant  Value=0.1
  q_out : Outport
  w_out : Outport  Port=2
  residual : Outport  Port=3
  bias estimat : Outport  Port=4
  wires:
  b(S)/1 -> Mux2/2
  R_sun(S)/1 -> Mux2/1
  Mux2/1 -> EKF/1
  R_sun(I)/1 -> Mux2/4
  b(I)/1 -> Mux2/5
  h_mw/1 -> Mux2/6
  N_mt/1 -> Mux2/7
  Clock/1 -> Mux2/8
  q0/1 -> Mux2/9
  Step size/1 -> Mux2/10
  Selector/1 -> q_out/1
  Eclipse/1 -> Mux2/11
  w(S)/1 -> Mux2/3
  EKF/1 -> Selector/1, Selector2/1, Selector1/1, Selector3/1
  Selector1/1 -> w_out/1
  Selector2/1 -> residual/1
  Selector3/1 -> bias estimat/1

== system components_lib/ADS/Attitude Determination/Propagator from Kalman filter ==
  q(S) : Inport  Port=1  LatchInput=off
  w(S) : Inport  Port=2  LatchInput=off
  h_mw(S) : Inport  Port=3  LatchInput=off
  N_mt(S) : Inport  Port=4  LatchInput=off
  N_dist(S) : Inport  Port=5  LatchInput=off
  Inertia matrix : Inport  Port=6  LatchInput=off
  EKF : MATLABFcn  MATLABFcn=kalman-propagator  OutputDimensions=10  SampleTime=1
  Mux2 : Mux  Inputs=7
  Selector : Selector  Elements=(1:4)  InputPortWidth=10
  Selector1 : Selector  Elements=(5:7)  InputPortWidth=10
  Selector2 : Selector  Elements=(8:10)  InputPortWidth=10
  Step size : Constant
  q_out : Outport
  w_out : Outport  Port=2
  h_mw : Outport  Port=3
  wires:
  Inertia matrix/1 -> Mux2/7
  N_mt(S)/1 -> Mux2/4
  Selector2/1 -> h_mw/1
  Selector1/1 -> w_out/1
  EKF/1 -> Selector1/1, Selector2/1, Selector/1
  h_mw(S)/1 -> Mux2/3
  Selector/1 -> q_out/1
  Step size/1 -> Mux2/6
  N_dist(S)/1 -> Mux2/5
  Mux2/1 -> EKF/1
  q(S)/1 -> Mux2/1
  w(S)/1 -> Mux2/2

== system components_lib/ADS/Attitude Determination/otoquest ==
  B (I) : Inport  Port=1  SampleTime=1  LatchInput=off
  R_sun(I) : Inport  Port=2  SampleTime=1  LatchInput=off
  B(S) : Inport  Port=3  SampleTime=1  LatchInput=off
  R_sun(S) : Inport  Port=4  SampleTime=1  LatchInput=off
  Mux : Mux  Inputs=6
  Weights : Constant  Value=[0.5,0.5]
  create q_old : UnitDelay  Orientation=left  X0=[0.8 0 0 0.6]
  otoquest.m : MATLABFcn  MATLABFcn=otoquest(u)  Output1D=off
  q(I->S) : Outport  PortDimensions=4
  wires:
  Weights/1 -> Mux/5
  R_sun(S)/1 -> Mux/4
  B(S)/1 -> Mux/3
  R_sun(I)/1 -> Mux/2
  B (I)/1 -> Mux/1
  otoquest.m/1 -> q(I->S)/1, create q_old/1
  Mux/1 -> otoquest.m/1
  create q_old/1 -> Mux/6

== system components_lib/ADS/Attitude Determination/otoquest with propagator ==
  B (I) : Inport  Port=1  SampleTime=1  LatchInput=off
  R_sun(I) : Inport  Port=2  SampleTime=1  LatchInput=off
  B(S) : Inport  Port=3  SampleTime=1  LatchInput=off
  R_sun(S) : Inport  Port=4  SampleTime=1  LatchInput=off
  omega : Inport  Port=5  SampleTime=1  LatchInput=off
  eclipse : Inport  Port=6  SampleTime=1  LatchInput=off
  Mux : Mux  Inputs=7
  Weights : Constant  Value=[0.5,0.5]
  otoquest.m : MATLABFcn  MATLABFcn=otoquest_with_pro(u)  Output1D=off  SampleTime=0.1
  q_p(I->S) : Outport  PortDimensions=4
  wires:
  omega/1 -> Mux/6
  eclipse/1 -> Mux/7
  Weights/1 -> Mux/5
  R_sun(S)/1 -> Mux/4
  B(S)/1 -> Mux/3
  R_sun(I)/1 -> Mux/2
  B (I)/1 -> Mux/1
  otoquest.m/1 -> q_p(I->S)/1
  Mux/1 -> otoquest.m/1

== system components_lib/ADS/Attitude Determination/q-method ==
  q(E->I) : Inport  Port=1  SampleTime=1  LatchInput=off
  R_s(I) : Inport  Port=2  SampleTime=1  LatchInput=off
  B(E) : Inport  Port=3  SampleTime=1  LatchInput=off
  B(sc) : Inport  Port=4  SampleTime=1  LatchInput=off
  R_s(sc) : Inport  Port=5  SampleTime=1  LatchInput=off
  Mux : Mux  Inputs=6
  Unit Delay : UnitDelay  Orientation=down
  Vector rotation by q : components_lib/Math utilities/Vector operations/Vector rotation by q
  Weights : Constant  Value=[1,0]
  qmethod.m : MATLABFcn  MATLABFcn=qmethod([u(1) u(4);u(2) u(5);u(3) u(6)] , [u(7) u(10);u(8) u(11); u(9) u(12)], [u(13);u(14)],[u(15);u(16);u(17);u(18)])  Output1D=off
  to unit vector{,1..3} (4 alike) : components_lib/Math utilities/Vector operations/to unit vector
  q(I-SC) : Outport  PortDimensions=4
  wires:
  qmethod.m/1 -> q(I-SC)/1, Unit Delay/1
  q(E->I)/1 -> Vector rotation by q/1
  B(E)/1 -> Vector rotation by q/2
  Mux/1 -> qmethod.m/1
  to unit vector/1 -> Mux/1
  to unit vector1/1 -> Mux/3
  Vector rotation by q/1 -> to unit vector1/1
  B(sc)/1 -> to unit vector/1
  R_s(I)/1 -> to unit vector3/1
  to unit vector3/1 -> Mux/4
  to unit vector2/1 -> Mux/2
  R_s(sc)/1 -> to unit vector2/1
  Unit Delay/1 -> Mux/6
  Weights/1 -> Mux/5

== system components_lib/ADS/FDI/Residual Generator ==
  Input : Inport  Port=1  LatchInput=off
  Measurement : Inport  Port=2  LatchInput=off
  A Matrix : Gain  Orientation=left  Gain=A  Multiplication=Matrix(K*u)
  B Matrix : Gain  Gain=B  Multiplication=Matrix(K*u)
  C Matrix : Gain  Gain=C  Multiplication=Matrix(K*u)
  Demux2 : Demux  Outputs=10
  Integrator : Integrator
  L Matrix : Gain  Orientation=left  Gain=L  Multiplication=Matrix(K*u)
  Q matrix : Gain  Gain=Q  Multiplication=Matrix(K*u)
  Scope5 : Scope  NumInputPorts=10
      settings: YMin=-5~0~0~-1.25e-009~-5e+028~0~0~-1~-1~-1  YMax=5~2e+028~5e+027~1~0~2e+028~5e+027~1~1~1  SaveName=ScopeData6
  Sum : Sum  Inputs=+++
  Sum1 : Sum  Inputs=|++
  Sum2 : Sum  Orientation=left  Inputs=+|-
  Working point : Constant  Value=[q_bar;w_bar; h_mw]
  residual : Outport
  wires:
  Input/1 -> B Matrix/1
  Q matrix/1 -> residual/1
  Working point/1 -> Sum1/2
  Measurement/1 -> Sum2/1
  C Matrix/1 -> Sum2/2, Demux2/1
  Sum2/1 -> L Matrix/1, Q matrix/1
  Sum1/1 -> C Matrix/1
  Integrator/1 -> Sum1/1, A Matrix/1
  Sum/1 -> Integrator/1
  A Matrix/1 -> Sum/3
  B Matrix/1 -> Sum/2
  L Matrix/1 -> Sum/1
  Demux2/1 -> Scope5/1
  Demux2/2 -> Scope5/2
  Demux2/3 -> Scope5/3
  Demux2/4 -> Scope5/4
  Demux2/5 -> Scope5/5
  Demux2/6 -> Scope5/6
  Demux2/7 -> Scope5/7
  Demux2/8 -> Scope5/8
  Demux2/9 -> Scope5/9
  Demux2/10 -> Scope5/10

== system components_lib/ADS/On-board model/ADS on-board models ==
  note: P_S - P_A
  note: R_sas
  note: R_s
  note: R_sa
  sim_time (JD) : Inport  Port=1  LatchInput=off
  Estimated q(I->S) : Inport  Port=2  LatchInput=off
  Albedo model onboard : Subsystem  AncestorBlock=components_lib/ADS/On-board Sensor model/Albedo model onboard  mask{sun_flux=1366.9, matrix=FOV cosine dep. reflectivity table, enable=off}
      mask prompts: sun_flux "Sun flux (mean: 1366.9)"; matrix "Choose used reflectivity data:"; enable "Use reflectivity matrix (blackbox)"
      mask init: same as components_lib/ADS/On-board model/Albedo model onboard
      mask StyleString: edit,popup(FOV cosine dep. reflectivity table|FOV meaned reflectivity table|Polynomial fit to latitude meaned reflectivity|Constant reflectivity of 30%),checkbox
  B to unit vector : components_lib/Math utilities/Vector operations/to unit vector
  Eclipse model : components_lib/ADS/On-board model/Eclipse model  r_e=6371010  theta_e=65
  Ephemeris on-board : components_lib/ADS/On-board model/Ephemeris on-board
  Orbit and Magnetic field models : components_lib/ADS/On-board model/Orbit and Magnetic field models  tle_type=Oersted TLE
  P_S - P_A to unit vector : components_lib/Math utilities/Vector operations/to unit vector
  Product : Product  Orientation=down  RndMeth=Zero
  R_sas flux to unit vector : components_lib/Math utilities/Vector operations/to unit vector
  R_sas to unit vector : components_lib/Math utilities/Vector operations/to unit vector
  "Solar flux [W/m^2] (1366.9) " : Constant  Orientation=down  Value=sun_flux
  Sum : Sum  Inputs=|-+
  Sum2 : Sum  Orientation=down  Inputs=|++
  "Sun vector rotation " : components_lib/Math utilities/Quaternion operations/Vector rotation by q
  Switch : Switch  Criteria=u2 ~= 0
  Zenith vector rotation : components_lib/Math utilities/Quaternion operations/Vector rotation by q
  albedo enabled : Constant  Value=alb_enabled
  Mag unit vector (I) : Outport
  Sun unit vector (I) : Outport  Port=2
  "Eclipse: 1=true, 0=false" : Outport  Port=3
  Albedo vector (I) : Outport  Port=4
  wires:
  albedo enabled/1 -> Switch/2
  Switch/1 -> Sun unit vector (I)/1
  Sum2/1 -> P_S - P_A to unit vector/1
  Product/1 -> Sum2/1, R_sas flux to unit vector/1
  Sum/1 -> R_sas to unit vector/1
  "Solar flux [W/m^2] (1366.9) "/1 -> Product/2
  R_sas to unit vector/1 -> Product/1
  Ephemeris on-board/2 -> "Sun vector rotation "/2, Eclipse model/1, Sum/2
  "Sun vector rotation "/1 -> Albedo model onboard/1("Earth -> Sun vector (ECEF)")
  Zenith vector rotation/1 -> Albedo model onboard/2(Zenith vector (ECEF))
  Orbit and Magnetic field models/2 -> Sum/1, Zenith vector rotation/2, Eclipse model/2
  Eclipse model/1 -> "Eclipse: 1=true, 0=false"/1
  Ephemeris on-board/1 -> "Sun vector rotation "/1, Zenith vector rotation/1, Albedo model onboard/4(q(I->E)), Orbit and Magnetic field models/2
  sim_time (JD)/1 -> Orbit and Magnetic field models/1, Ephemeris on-board/1
  Orbit and Magnetic field models/1 -> B to unit vector/1
  B to unit vector/1 -> Mag unit vector (I)/1
  P_S - P_A to unit vector/1 -> Switch/1
  R_sas flux to unit vector/1 -> Switch/3
  Estimated q(I->S)/1 -> Albedo model onboard/3(q(I->S))
  Albedo model onboard/1(Albedo vector (I)) -> Albedo vector (I)/1, Sum2/2  "alb_ob"
